simulink model "testSimBlocks"  (Simulink 7.4)
settings: Solver=ode45  StartTime=0.0  StopTime=10.0  MaxStep=0.01  RelTol=1e-3
values from neighbouring files (symbols this model uses):
  add1 = [1 1 1]    [testSimulinkBlocks.m]
  add2 = [1 2 2]    [testSimulinkBlocks.m]
  add3 = [1 2 3]    [testSimulinkBlocks.m]
  add4 = [9 9 9]    [testSimulinkBlocks.m]
settings Model: Creator=JJK  LastModifiedBy=JJK
settings DebuggingCC: SolverPrmCheckMsg=none

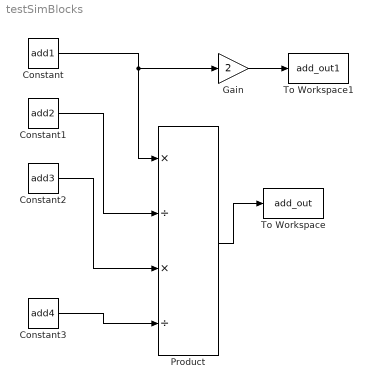
== system testSimBlocks ==
  Constant : Constant  Value=add1  OutDataType=fixdt(1, 16)  OutScaling=2^0
  Constant1 : Constant  Value=add2  OutDataType=fixdt(1, 16)  OutScaling=2^0
  Constant2 : Constant  Value=add3  OutDataType=fixdt(1, 16)  OutScaling=2^0
  Constant3 : Constant  Value=add4  OutDataType=fixdt(1, 16)  OutScaling=2^0
  Gain : Gain  Gain=2  ParameterDataType=fixdt(1, 16)  ParameterScaling=2^0  OutDataType=fixdt(1, 16)  OutScaling=2^0
  Product : Product  Inputs=*/*/  OutDataType=fixdt(1, 16)  OutScaling=2^0  RndMeth=Zero
  To Workspace : ToWorkspace  VariableName=add_out  SampleTime=-1  SaveFormat=Array
  To Workspace1 : ToWorkspace  VariableName=add_out1  SampleTime=-1  SaveFormat=Array
  wires:
  Constant/1 -> Product/1, Gain/1
  Constant1/1 -> Product/2
  Product/1 -> To Workspace/1
  Constant2/1 -> Product/3
  Constant3/1 -> Product/4
  Gain/1 -> To Workspace1/1
